simulink model "Active_Suspension_model"  (R2019a)
settings: Solver=ode15s  StartTime=0  StopTime=60  RelTol=1e-3  EnableMultiTasking=on
libraries: simulink x1
settings Model: Creator=Administrator  LastModifiedBy=Saismrithi Bhat
settings DataIOCC: SaveFormat=Array  ReturnWorkspaceOutputs=off
settings OptimizationCC: LifeSpan=inf
settings DebuggingCC: UnderspecifiedInitializationDetection=Classic  MergeDetectMultiDrivingBlocksExec=none  SolverPrmCheckMsg=warning  StateNameClashWarn=warning  SFUnexpectedBacktrackingDiag=warning  SFNoUnconditionalDefaultTransitionDiag=warning  SFExecutionAtInitializationDiag=none  ArithmeticOperatorsInVariantConditions=warning
settings HardwareCC: ProdBitPerPointer=32  ProdBitPerSizeT=32  ProdBitPerPtrDiffT=32  ProdLargestAtomicFloat=None  ProdIntDivRoundTo=Undefined  ProdEndianess=Unspecified  ProdWordSize=32  ProdHWDeviceType=32-bit Generic
settings ModelReferenceCC: PropagateSignalLabelsOutOfModel=off
settings SFSimCC: SimUseLocalCustomCode=off
settings RTWCC: RTWUseLocalCustomCode=off
settings CodeAppCC: StateflowObjectComments=on
settings GRTTargetCC: TargetLangStandard=C89/C90 (ANSI)  GeneratePreprocessorConditionals=Disable all
settings ConfigComp: CovMetricSettings=dw  CovHtmlReporting=on  CovSaveCumulativeToWorkspaceVar=on  CovSaveSingleToWorkspaceVar=on  CovExternalEMLEnable=off

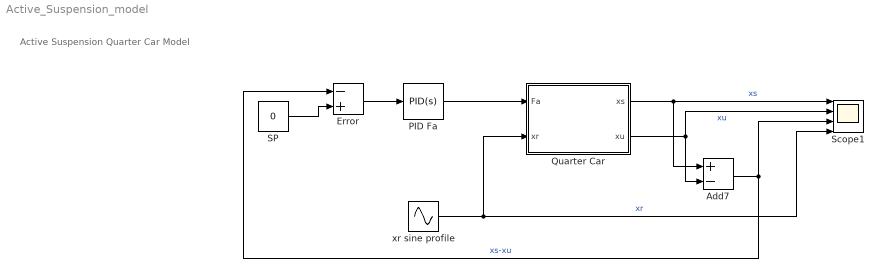
== system Active_Suspension_model ==
  note: Active Suspension Quarter Car Model
  Add7 : Sum  Inputs=+-
  Error : Sum  Inputs=-+
  PID Fa : simulink/Continuous/PID Controller  Controller=PID  Form=Parallel  TimeDomain=Continuous-time  SampleTime=1  IntegratorMethod=Forward Euler  FilterMethod=Forward Euler  ControllerParametersSource=internal  P=0  I=17490.1289315124  D=0  UseFilter=on  N=100  TunerSelectOption=Transfer Function Based (PID Tuner App)  InitialConditionSource=internal  InitialConditionForIntegrator=0  InitialConditionForFilter=0  DifferentiatorICPrevScaledInput=0  ExternalReset=none  TrackingMode=off  Kt=1  LimitOutput=on  UpperSaturationLimit=3000  LowerSaturationLimit=0  LinearizeAsGain=on  AntiWindupMode=none  Kb=1  POutMin=[]  POutMax=[]  IOutMin=[]  IOutMax=[]  DOutMin=[]  DOutMax=[]  NOutMin=[]  NOutMax=[]  SumOutMin=[]  SumOutMax=[]  SaturationOutMin=[]  SaturationOutMax=[]  PParamMin=[]  PParamMax=[]  IParamMin=[]  IParamMax=[]  DParamMin=[]  DParamMax=[]  NParamMin=[]  NParamMax=[]  KbParamMin=[]  KbParamMax=[]  KtParamMin=[]  KtParamMax=[]  KbOutMin=[]  KbOutMax=[]  KtOutMin=[]  KtOutMax=[]  IntegratorOutMin=[]  IntegratorOutMax=[]  FilterOutMin=[]  FilterOutMax=[]  SumI1OutMin=[]  SumI1OutMax=[]  SumI2OutMin=[]  SumI2OutMax=[]  SumI3OutMin=[]  SumI3OutMax=[]  SumI4OutMin=[]  SumI4OutMax=[]  SumDOutMin=[]  SumDOutMax=[]  DifferentiatorOutMin=[]  DifferentiatorOutMax=[]  FilterDiffOutCoefMin=[]  FilterDiffOutCoefMax=[]  ReciprocalOutMin=[]  ReciprocalOutMax=[]  SumDenOutMin=[]  SumDenOutMax=[]  SumNumOutMin=[]  SumNumOutMax=[]  DivideOutMin=[]  DivideOutMax=[]  IntegratorContinuousStateAttributes=''  IntegratorStateMustResolveToSignalObject=off  IntegratorRTWStateStorageClass=Auto  FilterContinuousStateAttributes=''  FilterStateMustResolveToSignalObject=off  FilterRTWStateStorageClass=Auto  ParallelPVariant=InternalParameters  IdealPVariant=Disabled  IVariant=InternalParameters  DVariant=InternalParameters  IntegratorVariant=Continuous  SatVariant=Enabled  AWVariant=Passthrough  PCopyVariant=Disabled  TRVariant=Disabled  FdbkBlocksVariant=Forward  IdealPFdbkVariant=Disabled  SatFdbkVariant=Disabled  DerivativeFilterVariant=ContFilter  NVariant=InternalParameters  NCopyVariant=Disabled  FilterICVariant=InternalICsFilter  IntegratorICVariant=InternalICs  ExternalResetVariant=Disabled  TRSumVariant=Passthrough  SumFdbkVariant=Disabled  SumVariant=Sum_PID
  Quarter Car : Subsystem
  SP : Constant  Value=0
  Scope1 : Scope  NumInputPorts=4
  xr sine profile : Sin  Amplitude=0.05  SampleTime=0
  wires:
  Error/1 -> PID Fa/1
  SP/1 -> Error/2
  Quarter Car/1(xs) -> Add7/1, Scope1/1  "xs"
  Quarter Car/2(xu) -> Scope1/2, Add7/2  "xu"
  xr sine profile/1 -> Scope1/4, Quarter Car/2(xr)  "xr"
  PID Fa/1 -> Quarter Car/1(Fa)
  Add7/1 -> Scope1/3, Error/1  "xs-xu"

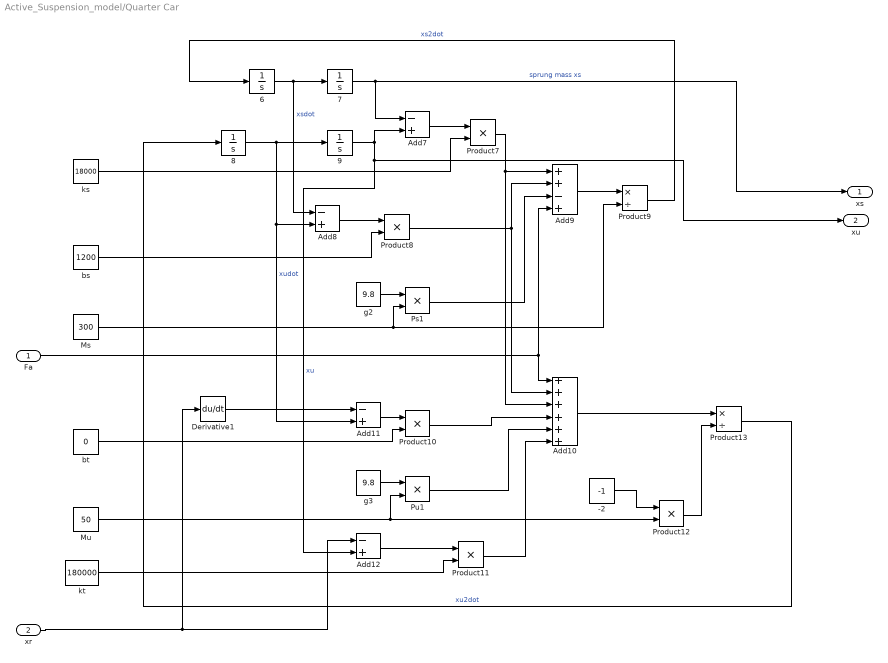
== system Active_Suspension_model/Quarter Car ==
  Fa : Inport
  xr : Inport  Port=2
  -2 : Constant  Value=-1
  {6..9} (4 alike) : Integrator
  Add10 : Sum  Inputs=++++++
  Add{7..8,11..12} (4 alike) : Sum  Inputs=-+
  Add9 : Sum  Inputs=++-+
  Derivative1 : Derivative
  Ms : Constant  Value=300
  Mu : Constant  Value=50
  Product{7..8,10..12} (5 alike) : Product
  Product13 : Product  Inputs=*/
  Product9 : Product  Inputs=*/
  Ps1 : Product
  Pu1 : Product
  bs : Constant  Value=1200
  bt : Constant  Value=0
  g2 : Constant  Value=9.8
  g3 : Constant  Value=9.8
  ks : Constant  Value=18000
  kt : Constant  Value=180000
  xs : Outport
  xu : Outport  Port=2
  wires:
  g2/1 -> Ps1/1
  Product12/1 -> Product13/2
  g3/1 -> Pu1/1
  Ps1/1 -> Add9/3
  Add10/1 -> Product13/1
  -2/1 -> Product12/1
  Mu/1 -> Pu1/2, Product12/2
  Product11/1 -> Add10/6
  Add12/1 -> Product11/1
  kt/1 -> Product11/2
  xr/1 -> Add12/1, Derivative1/1
  Pu1/1 -> Add10/5
  Product10/1 -> Add10/4
  Add11/1 -> Product10/1
  bt/1 -> Product10/2
  Derivative1/1 -> Add11/1
  Ms/1 -> Product9/2, Ps1/2
  Add9/1 -> Product9/1
  Fa/1 -> Add10/1, Add9/4
  Product8/1 -> Add10/2, Add9/2
  Product7/1 -> Add10/3, Add9/1
  bs/1 -> Product8/2
  Add8/1 -> Product8/1
  ks/1 -> Product7/2
  Add7/1 -> Product7/1
  9/1 -> Add12/2, xu/1, Add7/2  "xu"
  Product13/1 -> 8/1  "xu2dot"
  8/1 -> 9/1, Add8/2, Add11/2  "xudot"
  7/1 -> Add7/1, xs/1  "sprung mass xs"
  Product9/1 -> 6/1  "xs2dot"
  6/1 -> 7/1, Add8/1  "xsdot"
